simulink model "euler_ZXY_model"  (R2023b)
settings: Solver=FixedStepAuto  StartTime=0.0  StopTime=fs  FixedStep=ts  MaxStep=1e-4  RelTol=1e-3
undefined symbols (not defined in the file): alpha, alpha_1, alpha_2, alpha_d, e1, e2, e3, eta_0, eta_dot_0, f_max, g, gamma, gamma_d, gamma_e, gamma_u, gamma_x, gamma_x1, gamma_x2, J, k_3, k_beta, k_d_gamma, K_p, k_p_gamma, k_R, m, p_0, p_d_0, p_dot_0, p_dot_zmax, r, ts, y_c, z_c, z_dot_max, z_max
libraries: eeGeneralControl x8, slctrl_constraint x6, simulink x2, rbm3d x1, simulink_extras x1
(part 1 of 2)
settings Model: Creator=mori_keigo  LastModifiedBy=mori_keigo

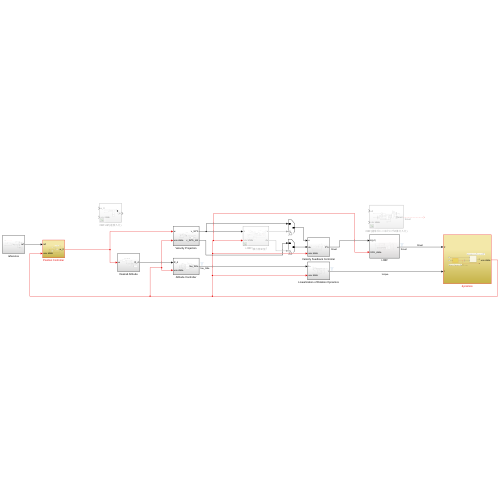
[thumbnail: Simulink's stored preview of the top-level diagram]
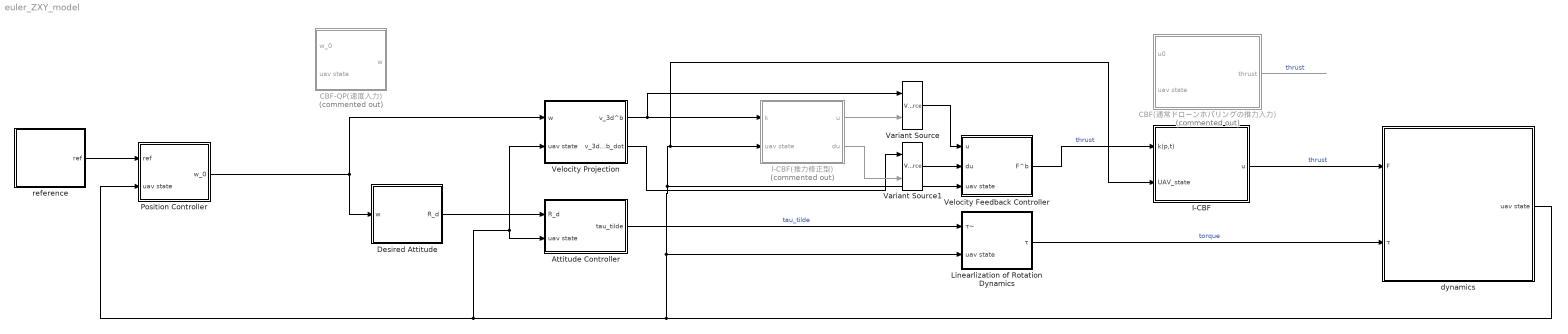
== system euler_ZXY_model ==
  Attitude Controller : Subsystem
  CBF(通常ドローンホバリングの推力入力) : Subsystem  Commented=on
  CBF-QP(速度入力) : Subsystem  Commented=on
  Desired Attitude : Subsystem
  I-CBF : Subsystem
  I-CBF(推力修正型) : Subsystem  Commented=on
  Linearlization of Rotation Dynamics : Subsystem
  Position Controller : Subsystem
  Variant Source : VariantSource
  Variant Source1 : VariantSource
  Velocity Feedback Controller : Subsystem
  Velocity Projection : Subsystem
  dynamics : Subsystem
  reference : Subsystem
  wires:
  Attitude Controller/1(tau_tilde) -> Linearlization of Rotation Dynamics/1(τ~)  "tau_tilde"
  Linearlization of Rotation Dynamics/1(τ) -> dynamics/2(τ)  "torque"
  Desired Attitude/1(R_d) -> Attitude Controller/1(R_d)
  reference/1(ref) -> Position Controller/1(ref)
  Velocity Feedback Controller/1(F^b) -> I-CBF/1(k(p,t))  "thrust"
  Position Controller/1(w_0) -> Desired Attitude/1(w), Velocity Projection/1(w)
  Velocity Projection/1(v_3d^b) -> Variant Source/1, I-CBF(推力修正型)/1(k)
  dynamics/1(uav state) -> I-CBF/2(UAV_state), I-CBF(推力修正型)/2(uav state), Velocity Feedback Controller/3(uav state), Linearlization of Rotation Dynamics/2(uav state), Velocity Projection/2(uav state), Attitude Controller/2(uav state), Position Controller/2(uav state)
  I-CBF(推力修正型)/1(u) -> Variant Source/2
  Velocity Projection/2(v_3d^b_dot) -> Variant Source1/1
  I-CBF(推力修正型)/2(du) -> Variant Source1/2
  Variant Source1/1 -> Velocity Feedback Controller/2(du)
  Variant Source/1 -> Velocity Feedback Controller/1(u)
  I-CBF/1(u) -> dynamics/1(F)  "thrust"
  CBF(通常ドローンホバリングの推力入力)/1(thrust) -> ?  "thrust"

== system euler_ZXY_model/Attitude Controller ==
  R_d : Inport
  Bus Element In1 : Inport  Port=2  PortName=uav state  Element=rotation.R_SO(2)
  Bus Element In2 : Inport  Port=2  PortName=uav state  Element=rotation.angle
  Bus Element In3 : Inport  Port=2  PortName=uav state  Element=rotation.velocity
  Constant : Constant  Value=0
  Selector : Selector  InputPortWidth=3  IndexOptions=Index vector (dialog)  Indices=[3]  OutputSizes=1
  Selector1 : Selector  InputPortWidth=3  IndexOptions=Index vector (dialog)  Indices=[3]  OutputSizes=1
  Selector2 : Selector  InputPortWidth=3  IndexOptions=Index vector (dialog)  Indices=[2]  OutputSizes=1
  Vector Concatenate : Concatenate  NumInputs=3
  beta_controller : Subsystem
  gamma_controller : Subsystem
  tau_tilde : Outport
  wires:
  beta_controller/1(tau_tilde_beta^b) -> Vector Concatenate/2
  gamma_controller/1(tau_tilde_gamma^b) -> Vector Concatenate/3
  Constant/1 -> Vector Concatenate/1
  Vector Concatenate/1 -> tau_tilde/1
  Bus Element In1/1 -> beta_controller/3(R_SO(2))
  Bus Element In2/1 -> Selector/1, Selector2/1
  Bus Element In3/1 -> Selector1/1
  Selector/1 -> gamma_controller/1(gamma)
  Selector1/1 -> gamma_controller/2(gamma_dot)
  Selector2/1 -> beta_controller/1(beta_dot)
  R_d/1 -> beta_controller/2(R_d)

== system euler_ZXY_model/CBF(通常ドローンホバリングの推力入力) ==
  u0 : Inport
  uav state : Inport  Port=2
  Bus Selector : BusSelector  OutputSignals=translation.position,translation.velocity,rotation.R,translation.lambda_1
  Constant : Constant  Value=0
  Constant1 : Constant  Value=0
  Constant2 : Constant  Value=0
  Constraint Enforcement : slctrl_constraint/Constraint Enforcement  nc=1  nu=1  c=0  external_c=on  external_umax=off  external_umin=on  Ts=0.1  maxiter=200  tol=1e-6  output_exitflag=on  relax_c=off  relax_u=off
      settings: LibrarySourceBlock=slctrlblks/Constraint Control/Constraint Enforcement
  MATLAB Function : MATLAB Function  TreatAsAtomicUnit=on
  Mux : Mux  Inputs=3
  Scope : Scope
  Scope1 : Scope
  Selector : Selector  InputPortWidth=3  IndexOptions=Index vector (dialog)  Indices=3  OutputSizes=1
  Selector1 : Selector  InputPortWidth=3  IndexOptions=Index vector (dialog)  Indices=3  OutputSizes=1
  Selector2 : Selector  InputPortWidth=3  IndexOptions=Index vector (dialog)  Indices=3  OutputSizes=1
  thrust : Outport
  wires:
  MATLAB Function/3(c) -> Constraint Enforcement/4
  MATLAB Function/2(gx) -> Constraint Enforcement/3
  MATLAB Function/1(fx) -> Constraint Enforcement/2
  uav state/1 -> Bus Selector/1
  Constant/1 -> Constraint Enforcement/5
  Bus Selector/3 -> MATLAB Function/3(rot)  "<R>"
  Bus Selector/4 -> MATLAB Function/4(lambda1)  "<lambda_1>"
  Constant2/1 -> Mux/2
  Constant1/1 -> Mux/1
  Constraint Enforcement/1 -> Scope1/1, Mux/3
  Mux/1 -> thrust/1
  Bus Selector/1 -> Selector/1  "<position>"
  Selector/1 -> MATLAB Function/1(z)
  Bus Selector/2 -> Selector1/1  "<velocity>"
  Selector1/1 -> MATLAB Function/2(z_dot)
  u0/1 -> Selector2/1
  Selector2/1 -> Constraint Enforcement/1
  Constraint Enforcement/2 -> Scope/1

== system euler_ZXY_model/CBF-QP(速度入力) ==
  w_0 : Inport
  In Bus Element : Inport  Port=2  PortName=uav state  Element=translation.position
  In Bus Element1 : Inport  Port=2  PortName=uav state  Element=rotation.angle
  Demux : Demux  Outputs=2
  ECBF-QP : Subsystem  Commented=on
  ECBF-QP_rengo_ver. : Subsystem
  ECBF-QP_z_only : Subsystem  Commented=on
  Scope : Scope
  Scope1 : Scope
  Scope2 : Scope
  Variant Source : VariantSource
  w : Outport
  wires:
  In Bus Element1/1 -> ECBF-QP_rengo_ver./3(eta)
  In Bus Element/1 -> ECBF-QP_rengo_ver./2(p)
  ECBF-QP_rengo_ver./1(Out1) -> Variant Source/2
  w_0/1 -> ECBF-QP_rengo_ver./1(w0), Variant Source/1
  Variant Source/1 -> Demux/1, Scope/1, w/1
  Demux/1 -> Scope2/1
  Demux/2 -> Scope1/1

== system euler_ZXY_model/Desired Attitude ==
  note: $R_d = \left [ (-1)^{\^} \frac{u}{||u||} \quad \frac{u}{||u||} \right ]$
  w : Inport
  Acos : Trigonometry  Operator=asin
  Display : Display
  Mux : Mux  Inputs=3
  Selector1 : Selector  NumberOfDimensions=2  InputPortWidth=3  IndexOptions=Index vector (dialog),Index vector (dialog)  Indices=[2],[1]  OutputSizes=1,1
  Terminator : Terminator
  alpha_d : Constant  Value=alpha_d
  desired attitude : Subsystem
  gamma_d : Constant  Value=gamma_d
  R_d : Outport
  wires:
  w/1 -> desired attitude/1(w)
  alpha_d/1 -> Mux/1
  Acos/1 -> Mux/2
  Selector1/1 -> Acos/1
  gamma_d/1 -> Mux/3
  Mux/1 -> Terminator/1, Display/1  "desired_attitude"
  desired attitude/1(R_d) -> Selector1/1, R_d/1

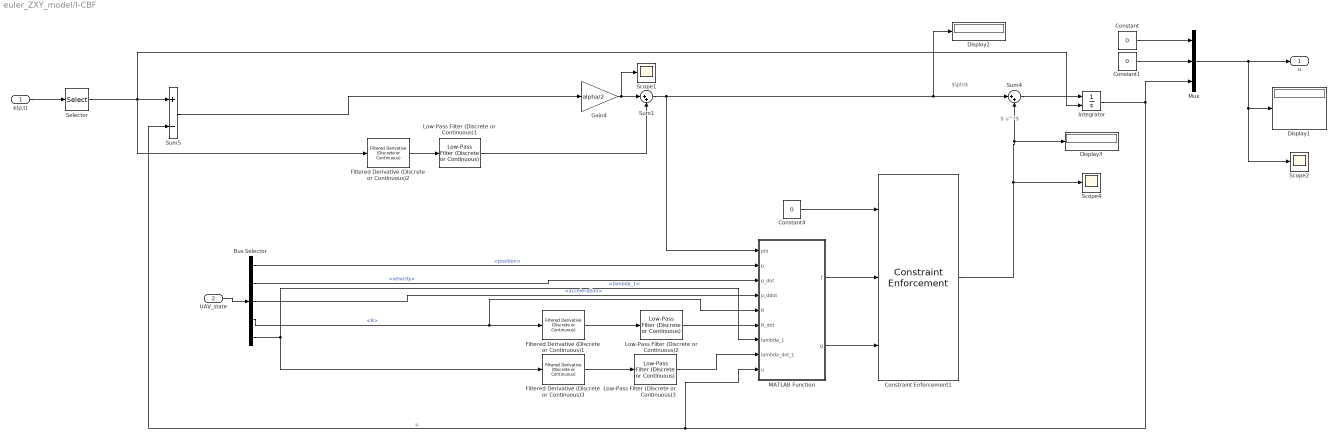
== system euler_ZXY_model/I-CBF ==
  note: $\nu^*$
  note: $\phi$
  k(p,t) : Inport
  UAV_state : Inport  Port=2
  Bus Selector : BusSelector  OutputSignals=translation.position,translation.velocity,translation.acceleration,rotation.R,translation.lambda_1
  Constant : Constant  Value=0
  Constant1 : Constant  Value=0
  Constant4 : Constant  Value=0
  Constraint Enforcement1 : slctrl_constraint/Constraint Enforcement  nc=2  nu=1  c=[0;0]  external_c=off  external_umax=off  external_umin=off  Ts=ts  maxiter=200  tol=1e-6  output_exitflag=on  relax_c=off  relax_u=off
      settings: LibrarySourceBlock=slctrlblks/Constraint Control/Constraint Enforcement
  Display1 : Display
  Display2 : Display
  Display3 : Display
  Filtered Derivative (Discrete or Continuous)1 : eeGeneralControl/Filtered Derivative (Discrete or Continuous)  K=1  T=0.1  B=inf  A=-inf  minRatio=10  init_option=Inherited from block input  x0=0  Ts=-1
      settings: LibrarySourceBlock=|
      | ee_sl_lib/General Control/Filtered Derivative
      | (Discrete or Continuous)
  Filtered Derivative (Discrete or Continuous)2 : eeGeneralControl/Filtered Derivative (Discrete or Continuous)  K=1  T=0.1  B=inf  A=-inf  minRatio=10  init_option=Inherited from block input  x0=0  Ts=-1
      settings: LibrarySourceBlock=|
      | ee_sl_lib/General Control/Filtered Derivative
      | (Discrete or Continuous)
  Filtered Derivative (Discrete or Continuous)3 : eeGeneralControl/Filtered Derivative (Discrete or Continuous)  K=1  T=0.1  B=inf  A=-inf  minRatio=10  init_option=Inherited from block input  x0=0  Ts=-1
      settings: LibrarySourceBlock=|
      | ee_sl_lib/General Control/Filtered Derivative
      | (Discrete or Continuous)
  Gain4 : Gain  Gain=alpha/2
  Integrator : Integrator  InitialConditionSource=external  InitialCondition=5
  Low-Pass Filter (Discrete or Continuous)1 : eeGeneralControl/Low-Pass Filter (Discrete or Continuous)  K=1  T=0.5  B=inf  A=-inf  init_option=Inherited from block input  x0=0  Ts=-1
  Low-Pass Filter (Discrete or Continuous)2 : eeGeneralControl/Low-Pass Filter (Discrete or Continuous)  K=1  T=0.5  B=inf  A=-inf  init_option=Inherited from block input  x0=0  Ts=-1
  Low-Pass Filter (Discrete or Continuous)3 : eeGeneralControl/Low-Pass Filter (Discrete or Continuous)  K=1  T=0.5  B=inf  A=-inf  init_option=Inherited from block input  x0=0  Ts=-1
  MATLAB Function : MATLAB Function  TreatAsAtomicUnit=on
  Mux : Mux  Inputs=3
  Scope1 : Scope
  Scope2 : Scope
  Scope4 : Scope
  Selector : Selector  InputPortWidth=3  IndexOptions=Index vector (dialog)  Indices=3  OutputSizes=1
  Sum1 : Sum  Inputs=|++
  Sum4 : Sum  Inputs=|++
  Sum5 : Sum  Inputs=+-
  u : Outport
  wires:
  UAV_state/1 -> Bus Selector/1
  Sum4/1 -> Integrator/1
  Constraint Enforcement1/1 -> Sum4/2, Display3/1, Scope4/1
  Sum1/1 -> MATLAB Function/1(phi), Display2/1, Sum4/1
  Gain4/1 -> Scope1/1, Sum1/1
  Sum5/1 -> Gain4/1
  Bus Selector/2 -> MATLAB Function/3(p_dot)  "<velocity>"
  Bus Selector/3 -> MATLAB Function/4(p_ddot)  "<acceleration>"
  Constant4/1 -> Constraint Enforcement1/1
  MATLAB Function/1(f) -> Constraint Enforcement1/2
  MATLAB Function/2(g) -> Constraint Enforcement1/3
  Bus Selector/4 -> Filtered Derivative (Discrete or Continuous)1/1, MATLAB Function/5(R)  "<R>"
  Bus Selector/1 -> MATLAB Function/2(p)  "<position>"
  Integrator/1 -> MATLAB Function/9(u), Sum5/2, Mux/3  "u"
  Bus Selector/5 -> MATLAB Function/7(lambda_1), Filtered Derivative (Discrete or Continuous)3/1  "<lambda_1>"
  k(p,t)/1 -> Selector/1
  Selector/1 -> Integrator/2, Sum5/1, Filtered Derivative (Discrete or Continuous)2/1
  Mux/1 -> Scope2/1, Display1/1, u/1
  Constant1/1 -> Mux/2
  Constant/1 -> Mux/1
  Filtered Derivative (Discrete or Continuous)2/1 -> Low-Pass Filter (Discrete or Continuous)1/1
  Low-Pass Filter (Discrete or Continuous)1/1 -> Sum1/2
  Low-Pass Filter (Discrete or Continuous)2/1 -> MATLAB Function/6(R_dot)
  Filtered Derivative (Discrete or Continuous)1/1 -> Low-Pass Filter (Discrete or Continuous)2/1
  Filtered Derivative (Discrete or Continuous)3/1 -> Low-Pass Filter (Discrete or Continuous)3/1
  Low-Pass Filter (Discrete or Continuous)3/1 -> MATLAB Function/8(lambda_dot_1)

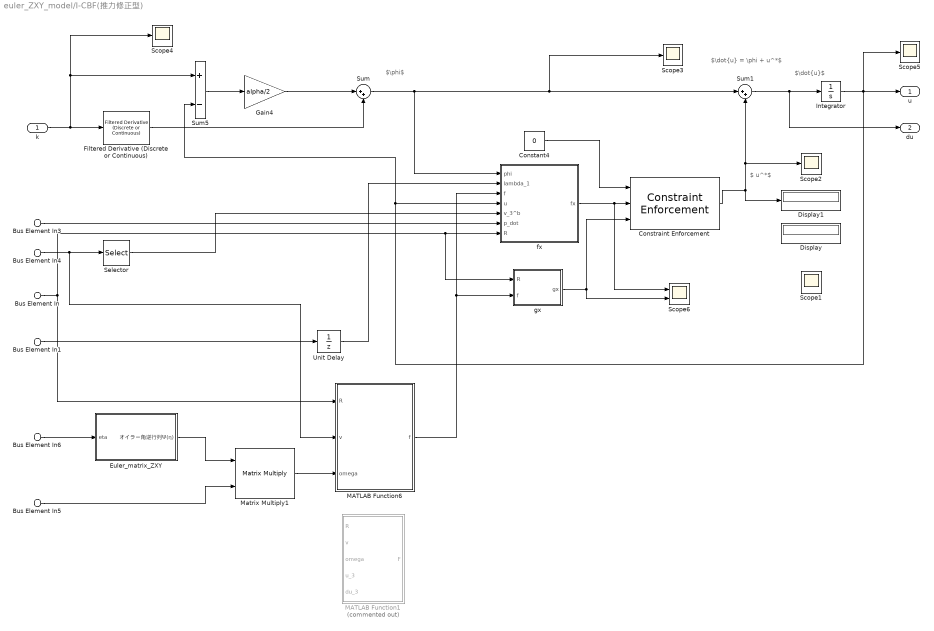
== system euler_ZXY_model/I-CBF(推力修正型) ==
  note: $\dot{u}$
  note: $\dot{u} = \phi + \nu^*$
  note: $\phi$
  note: $\nu^*$
  k : Inport
  Bus Element In : Inport  Port=2  PortName=uav state  Element=rotation.R
  Bus Element In5 : Inport  Port=2  PortName=uav state  Element=rotation.velocity
  Bus Element In6 : Inport  Port=2  PortName=uav state  Element=rotation.angle
  Bus Element In1 : Inport  Port=2  PortName=uav state  Element=translation.lambda_1
  Bus Element In3 : Inport  Port=2  PortName=uav state  Element=translation.velocity
  Bus Element In4 : Inport  Port=2  PortName=uav state  Element=translation.body_velocity
  Constant4 : Constant  Value=0
  Constraint Enforcement : slctrl_constraint/Constraint Enforcement  nc=1  nu=1  c=0  external_c=off  external_umax=off  external_umin=off  Ts=ts  maxiter=200  tol=1e-6  output_exitflag=on  relax_c=off  relax_u=off
      settings: LibrarySourceBlock=slctrlblks/Constraint Control/Constraint Enforcement
  Display : Display
  Display1 : Display
  Euler_matrix_ZXY : Subsystem
  Filtered Derivative (Discrete or Continuous) : eeGeneralControl/Filtered Derivative (Discrete or Continuous)  K=1  T=0.1  B=inf  A=-inf  minRatio=10  init_option=Inherited from block input  x0=0  Ts=-1
      settings: LibrarySourceBlock=|
      | ee_sl_lib/General Control/Filtered Derivative
      | (Discrete or Continuous)
  Gain4 : Gain  Gain=alpha/2
  Integrator : Integrator
  MATLAB Function1 : MATLAB Function  Commented=on  TreatAsAtomicUnit=on
  MATLAB Function6 : MATLAB Function  TreatAsAtomicUnit=on
  Matrix Multiply1 : Product  Multiplication=Matrix(*)
  Scope{1..5} (5 alike) : Scope
  Scope6 : Scope  NumInputPorts=2
  Selector : Selector  InputPortWidth=3  IndexOptions=Index vector (dialog)  Indices=3  OutputSizes=1
  Sum : Sum  Inputs=|++
  Sum1 : Sum  Inputs=|++
  Sum5 : Sum  Inputs=+-
  Unit Delay : UnitDelay  SampleTime=-1  HasFrameUpgradeWarning=on
  fx : Subsystem
  gx : Subsystem
  u : Outport
  du : Outport  Port=2
  wires:
  Integrator/1 -> Scope5/1, u/1, Sum5/2, fx/4(u)
  Constraint Enforcement/1 -> Sum1/2, Scope2/1, Display1/1
  Sum/1 -> fx/1(phi), Scope3/1, Sum1/1
  Gain4/1 -> Sum/1
  Sum5/1 -> Gain4/1
  Constant4/1 -> Constraint Enforcement/1
  ? -> Scope1/1, Display/1
  Sum1/1 -> du/1, Integrator/1
  fx/1(fx) -> Scope6/1, Constraint Enforcement/2
  gx/1(gx) -> Constraint Enforcement/3, Scope6/2
  k/1 -> Filtered Derivative (Discrete or Continuous)/1, Scope4/1, Sum5/1
  Filtered Derivative (Discrete or Continuous)/1 -> Sum/2
  Bus Element In/1 -> gx/1(R), fx/7(R), MATLAB Function6/1(R)
  MATLAB Function6/1(f) -> fx/3(f), gx/2(f)
  Bus Element In5/1 -> Matrix Multiply1/2
  Bus Element In6/1 -> Euler_matrix_ZXY/1(eta)
  Euler_matrix_ZXY/1(オイラー角逆行列Ψ(η)) -> Matrix Multiply1/1
  Matrix Multiply1/1 -> MATLAB Function6/3(omega)
  Bus Element In4/1 -> MATLAB Function6/2(v), Selector/1
  Selector/1 -> fx/5(v_3^b)
  Bus Element In3/1 -> fx/6(p_dot)
  Bus Element In1/1 -> Unit Delay/1
  Unit Delay/1 -> fx/2(lambda_1)

== system euler_ZXY_model/Linearlization of Rotation Dynamics ==
  τ~ : Inport
  Bus Element In1 : Inport  Port=2  PortName=uav state  Element=rotation.Psi
  Bus Element In2 : Inport  Port=2  PortName=uav state  Element=rotation.lambda_3
  Bus Element In3 : Inport  Port=2  PortName=uav state  Element=rotation.velocity
  Constant : Constant  Value=J  VectorParams1D=off
  Constant1 : Constant  Value=e1
  Product : Product  Inputs=3  Multiplication=Matrix(*)
  Product1 : Product  Inputs=/  Multiplication=Matrix(*)
  Product2 : Product  Inputs=3  Multiplication=Matrix(*)
  Product3 : Product  Multiplication=Matrix(*)
  Scope : Scope
  Sum : Sum  Inputs=|+++
  Transpose1 : Math  Operator=transpose
  Unit Delay : UnitDelay  SampleTime=-1  HasFrameUpgradeWarning=on
  τ : Outport
  wires:
  τ~/1 -> Scope/1, Product/3
  Constant/1 -> Product/1
  Product/1 -> Sum/1
  Product2/1 -> Sum/2
  Sum/1 -> τ/1
  Bus Element In1/1 -> Transpose1/1, Product/2
  Transpose1/1 -> Product1/1
  Constant1/1 -> Product3/1
  Product3/1 -> Sum/3
  Bus Element In2/1 -> Unit Delay/1
  Unit Delay/1 -> Product3/2
  Product1/1 -> Product2/1
  [C] -> Product2/2
  Bus Element In3/1 -> Product2/3

== system euler_ZXY_model/Position Controller ==
  note: $w_0 = - K_p ~ p_e + \dot{p}_d$
  Bus Element In : Inport  PortName=ref  Element=position
  Bus Element In1 : Inport  PortName=ref  Element=velocity
  In Bus Element : Inport  Port=2  PortName=uav state  Element=translation.position
  Constant : Constant  Value=K_p
  Matrix Multiply : Product  Multiplication=Matrix(*)
  Selector : Selector  InputPortWidth=3  IndexOptions=Index vector (dialog)  Indices=[2 3]  OutputSizes=1
  Sum : Sum  Inputs=|+-
  Sum1 : Sum  Inputs=|++
  w_0 : Outport
  wires:
  Bus Element In/1 -> Sum/1
  Matrix Multiply/1 -> Sum1/1
  Constant/1 -> Matrix Multiply/1
  Sum/1 -> Matrix Multiply/2
  Sum1/1 -> w_0/1
  Bus Element In1/1 -> Sum1/2
  In Bus Element/1 -> Selector/1
  Selector/1 -> Sum/2

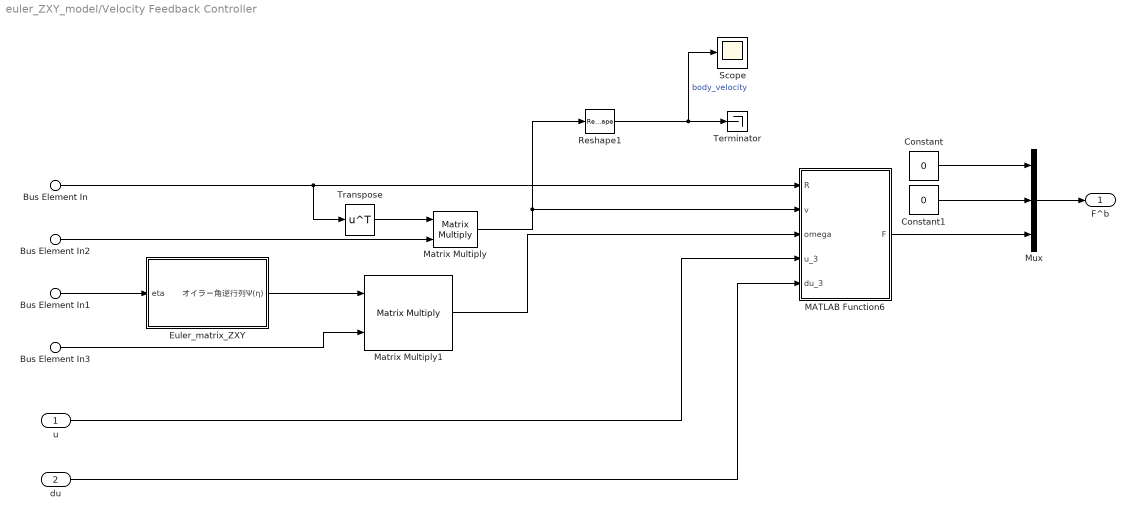
== system euler_ZXY_model/Velocity Feedback Controller ==
  u : Inport
  du : Inport  Port=2
  Bus Element In3 : Inport  Port=3  PortName=uav state  Element=rotation.velocity
  Bus Element In1 : Inport  Port=3  PortName=uav state  Element=rotation.angle
  Bus Element In : Inport  Port=3  PortName=uav state  Element=rotation.R
  Bus Element In2 : Inport  Port=3  PortName=uav state  Element=translation.velocity
  Constant : Constant  Value=0
  Constant1 : Constant  Value=0
  Euler_matrix_ZXY : Subsystem
  MATLAB Function6 : MATLAB Function  TreatAsAtomicUnit=on
  Matrix Multiply : Product  Multiplication=Matrix(*)
  Matrix Multiply1 : Product  Multiplication=Matrix(*)
  Mux : Mux  Inputs=3
  Reshape1 : Reshape
  Scope : Scope
  Terminator : Terminator
  Transpose : Math  Operator=transpose
  F^b : Outport
  wires:
  u/1 -> MATLAB Function6/4(u_3)
  Transpose/1 -> Matrix Multiply/1
  Bus Element In2/1 -> Matrix Multiply/2
  Bus Element In/1 -> MATLAB Function6/1(R), Transpose/1
  Matrix Multiply1/1 -> MATLAB Function6/3(omega)
  Matrix Multiply/1 -> Reshape1/1, MATLAB Function6/2(v)
  Reshape1/1 -> Scope/1, Terminator/1  "body_velocity"
  Bus Element In3/1 -> Matrix Multiply1/2
  Euler_matrix_ZXY/1(オイラー角逆行列Ψ(η)) -> Matrix Multiply1/1
  Bus Element In1/1 -> Euler_matrix_ZXY/1(eta)
  MATLAB Function6/1(F) -> Mux/3
  Mux/1 -> F^b/1
  Constant1/1 -> Mux/2
  Constant/1 -> Mux/1
  du/1 -> MATLAB Function6/5(du_3)

== system euler_ZXY_model/Velocity Projection ==
  note: $v_z = u^T Re_2$
  w : Inport
  In Bus Element : Inport  Port=2  PortName=uav state  Element=rotation.R_SO(2)
  Constant : Constant  Value=[0;1]  VectorParams1D=off
  Filtered Derivative (Discrete or Continuous)2 : eeGeneralControl/Filtered Derivative (Discrete or Continuous)  K=1  T=0.1  B=inf  A=-inf  minRatio=10  init_option=Inherited from block input  x0=0  Ts=-1
      settings: LibrarySourceBlock=|
      | ee_sl_lib/General Control/Filtered Derivative
      | (Discrete or Continuous)
  Matrix Multiply : Product  Inputs=3  Multiplication=Matrix(*)
  Transpose : Math  Operator=transpose
  v_3d^b : Outport
  v_3d^b_dot : Outport  Port=2
  wires:
  In Bus Element/1 -> Matrix Multiply/2
  Transpose/1 -> Matrix Multiply/1
  Matrix Multiply/1 -> Filtered Derivative (Discrete or Continuous)2/1, v_3d^b/1
  w/1 -> Transpose/1
  Constant/1 -> Matrix Multiply/3
  Filtered Derivative (Discrete or Continuous)2/1 -> v_3d^b_dot/1

== system euler_ZXY_model/dynamics ==
  note: $m \ddot{p} + mg e_3 + \lambda_1 A^T + \lambda_2 e_1 = RF^b$
  note: $M(\eta) \ddot{\eta} + C(\eta,\dot{\eta}) \dot{\eta} = \Psi(\eta)^T \tau^b - \lambda_3 e_1$
  F : Inport
  τ : Inport  Port=2
  Bus Selector : BusSelector  OutputSignals=angle
  並進方向の運動方程式 : Subsystem
  回転方向の運動方程式 : Subsystem
  Bus Element Out1 : Outport  PortName=uav state  Element=translation
  Bus Element Out : Outport  PortName=uav state  Element=rotation
  wires:
  τ/1 -> 回転方向の運動方程式/1(τ^b)
  F/1 -> 並進方向の運動方程式/1(F_b)
  並進方向の運動方程式/1(translation) -> Bus Element Out1/1
  回転方向の運動方程式/1(attitude_state) -> Bus Selector/1, Bus Element Out/1
  Bus Selector/1 -> 並進方向の運動方程式/2(eta)  "<angle>"

== system euler_ZXY_model/reference ==
  Clock1 : Clock
  Constant : Constant  Value=0.20
  Constant1 : Constant  Value=0
  Constant2 : Constant  Commented=on  Value=0
  Demux : Demux  Outputs=2
  Integrator : Integrator  InitialCondition=p_d_0
  Mux : Mux  Inputs=2
  Mux1 : Mux  Inputs=2
  Terminator : Terminator
  XY Graph : Record  FileSettingsInternal="{\"entries\":[{\"content\":{\"excelSettings\":{\"content\":{},\"type\":\"Streamout.ExcelSettings\"}},\"type\":\"Streamout.FileSettingStorage\",\"uuid\":\"\"}],\"packageUris\":[\"http:\\/\\/schema.mathworks.com\\/mf0\\/streamout_blocks\\/R2020a\"],\"version\":\"1.0\"}"  Layout=[1 1]  SignalsInternal="{\"entries\":[{\"content\":{\"signals\":[{\"content\":{\"blockPath\":[],\"dimensions\":[1],\"domain\":\"\",\"lineColor\":\"#edb120\",\"port\":1,\"signalID\":8,\"signalName\":\"Demux:1\"},\"type\":\"RecordBlkView.Signal\",\"uuid\":\"\"},{\"content\":{\"blockPath\":[],\"dimensions\":[1],\"domain\":\"\",\"lineColor\":\"#7e2f8e\",\"port\":2,\"signalID\":11,\"signalName\":\"Demux:2\"},\"type\":\"RecordBlkView.Signal\",\"uuid\":\"\"}]},\"type\":\"RecordBlkView.InputSignals\",\"uuid\":\"\"}],\"packageUris\":[\"http:\\/\\/schema.mathworks.com\\/mf0\\/streamout_blocks\\/R2020a\"],\"version\":\"1.0\"}"  VisualizationBindings="{\"xyplotplugin\":{\"info\":[{\"series\":[],\"subplotID\":1}]}}"  CompatibilityTag=XY
  y_d_dot : Stateflow chart  TreatAsAtomicUnit=on
  Out Bus Element : Outport  PortName=ref  Element=position
  Out Bus Element1 : Outport  PortName=ref  Element=velocity
  wires:
  Clock1/1 -> y_d_dot/1(t)
  Constant/1 -> Mux/2
  y_d_dot/1(y_d_dot) -> Mux/1
  Mux/1 -> Out Bus Element1/1, Integrator/1
  Demux/1 -> XY Graph/1
  Demux/2 -> XY Graph/2
  Integrator/1 -> Mux1/2, Out Bus Element/1, Demux/1
  Constant1/1 -> Mux1/1
  Mux1/1 -> Terminator/1  "p_d"
  Constant2/1 -> ?

== system euler_ZXY_model/Attitude Controller/beta_controller ==
  beta_dot : Inport
  R_d : Inport  Port=2
  R_SO(2) : Inport  Port=3
  Derivative : Derivative  Commented=on
  Discrete Derivative : simulink/Discrete/Discrete Derivative  gainval=1.0  ICPrevScaledInput=0.0  OutMin=[]  OutMax=[]  OutDataType=fixdt(1, 16)  OutScaling=2^-10  DoSatur=off
  Gain : Gain  Gain=-k_beta
  Scope : Scope
  Scope1 : Scope
  Sum : Sum  Inputs=|+-
  Sum1 : Sum  Inputs=|++
  r_beta : Subsystem
  tau_tilde_beta^b : Outport
  wires:
  beta_dot/1 -> Sum/1
  Gain/1 -> Sum1/1
  Sum1/1 -> Scope1/1, tau_tilde_beta^b/1
  r_beta/1(r_beta) -> Discrete Derivative/1, Sum/2
  Sum/1 -> Scope/1, Gain/1
  Discrete Derivative/1 -> Sum1/2
  R_d/1 -> r_beta/1(R_d)
  R_SO(2)/1 -> r_beta/2(R_SO(2))

== system euler_ZXY_model/Attitude Controller/gamma_controller ==
  gamma : Inport
  gamma_dot : Inport  Port=2
  Constant : Constant  Value=gamma_d
  Derivative : Derivative
  Gain : Gain  Gain=-k_p_gamma
  Gain1 : Gain  Gain=-k_d_gamma
  Sum : Sum  Inputs=|++
  Sum1 : Sum  Inputs=|-+
  Sum2 : Sum  Inputs=|-+
  tau_tilde_gamma^b : Outport
  wires:
  Sum/1 -> tau_tilde_gamma^b/1
  Gain/1 -> Sum/1
  Gain1/1 -> Sum/2
  Constant/1 -> Derivative/1, Sum1/1
  Sum2/1 -> Gain1/1
  Derivative/1 -> Sum2/1
  Sum1/1 -> Gain/1
  gamma/1 -> Sum1/2
  gamma_dot/1 -> Sum2/2

== system euler_ZXY_model/CBF-QP(速度入力)/ECBF-QP ==
  u0 : Inport
  p : Inport  Port=2
  eta : Inport  Port=3
  p_dot : Inport  Port=4
  body_velocity : Inport  Port=5
  eta_dot : Inport  Port=6
  Constraint Enforcement : slctrl_constraint/Constraint Enforcement  nc=1  nu=2  c=0  external_c=on  external_umax=off  external_umin=off  Ts=0.01  maxiter=200  tol=1e-6  output_exitflag=off  relax_c=off  relax_u=off
  Scope : Scope
  Scope1 : Scope
  Subsystem : Subsystem
  c : Subsystem
  gx : Subsystem
  Out1 : Outport
  wires:
  u0/1 -> Constraint Enforcement/1, Scope/1
  p/1 -> Subsystem/1(p), gx/1(p), c/1(p)
  eta/1 -> Subsystem/3(eta), gx/2(eta)
  Subsystem/1(fx) -> Constraint Enforcement/2
  gx/1(gx) -> Constraint Enforcement/3
  c/1(c) -> Constraint Enforcement/4
  Constraint Enforcement/1 -> Scope1/1, Out1/1
  p_dot/1 -> Subsystem/2(p_dot), c/2(p_dot)
  body_velocity/1 -> Subsystem/4(body_velocity)
  eta_dot/1 -> Subsystem/5(eta_dot)

== system euler_ZXY_model/CBF-QP(速度入力)/ECBF-QP_rengo_ver. ==
  w0 : Inport
  p : Inport  Port=2
  eta : Inport  Port=3
  Constraint Enforcement : slctrl_constraint/Constraint Enforcement  nc=1  nu=2  c=0  external_c=on  external_umax=off  external_umin=off  Ts=0.01  maxiter=200  tol=1e-6  output_exitflag=off  relax_c=off  relax_u=off
  Scope : Scope
  Scope1 : Scope
  c : Subsystem
  fx : Constant  Value=0  VectorParams1D=off
  gx : Subsystem
  Out1 : Outport
  wires:
  w0/1 -> Scope/1, Constraint Enforcement/1
  p/1 -> c/1(p), gx/1(p)
  eta/1 -> gx/2(eta), c/2(eta)
  fx/1 -> Constraint Enforcement/2
  gx/1(gx) -> Constraint Enforcement/3
  c/1(c) -> Constraint Enforcement/4
  Constraint Enforcement/1 -> Scope1/1, Out1/1

== system euler_ZXY_model/CBF-QP(速度入力)/ECBF-QP_z_only ==
  u0 : Inport
  p : Inport  Port=2
  eta : Inport  Port=3
  p_dot : Inport  Port=4
  body_velocity : Inport  Port=5
  eta_dot : Inport  Port=6
  Constraint Enforcement : slctrl_constraint/Constraint Enforcement  nc=1  nu=2  c=0  external_c=on  external_umax=off  external_umin=off  Ts=0.01  maxiter=200  tol=1e-6  output_exitflag=off  relax_c=off  relax_u=off
  Scope : Scope
  Scope1 : Scope
  Subsystem : Subsystem
  c : Subsystem
  gx : Subsystem
  Out1 : Outport
  wires:
  u0/1 -> Constraint Enforcement/1, Scope/1
  p/1 -> c/1(p)
  eta/1 -> Subsystem/1(eta), gx/1(eta)
  Subsystem/1(fx) -> Constraint Enforcement/2
  gx/1(gx) -> Constraint Enforcement/3
  c/1(c) -> Constraint Enforcement/4
  Constraint Enforcement/1 -> Scope1/1, Out1/1
  p_dot/1 -> c/2(p_dot)
  body_velocity/1 -> Subsystem/2(body_velocity)
  eta_dot/1 -> Subsystem/3(eta_dot)

== system euler_ZXY_model/Desired Attitude/desired attitude ==
  w : Inport
  (-1)^ : Constant  Value=[0 1; -1 0]  VectorParams1D=off
  Divide : Product  Inputs=*/
  Dot Product : DotProduct  OutDataTypeStr=Inherit: Inherit via internal rule
  Matrix Concatenate : Concatenate  Mode=Multidimensional array  ConcatenateDimension=2
  Matrix Multiply : Product  Multiplication=Matrix(*)
  Square Root : Sqrt
  R_d : Outport
  wires:
  Dot Product/1 -> Square Root/1
  w/1 -> Divide/1, Dot Product/2, Dot Product/1
  Square Root/1 -> Divide/2
  Matrix Concatenate/1 -> R_d/1
  Divide/1 -> Matrix Concatenate/2, Matrix Multiply/2
  (-1)^/1 -> Matrix Multiply/1
  Matrix Multiply/1 -> Matrix Concatenate/1

== system euler_ZXY_model/I-CBF(推力修正型)/Euler_matrix_ZXY ==
  eta : Inport
  Constant : Constant  Value=e2
  Matrix Concatenate4 : Concatenate  NumInputs=3  Mode=Multidimensional array  ConcatenateDimension=2
  Psi_*1 : Subsystem
  Psi_*2 : Subsystem
  オイラー角逆行列Ψ(η) : Outport  VectorParamsAs1DForOutWhenUnconnected=off
  wires:
  eta/1 -> Psi_*1/1(eta), Psi_*2/1(eta)
  Matrix Concatenate4/1 -> オイラー角逆行列Ψ(η)/1
  Psi_*2/1(Out1) -> Matrix Concatenate4/2
  Psi_*1/1(Out1) -> Matrix Concatenate4/1
  Constant/1 -> Matrix Concatenate4/3

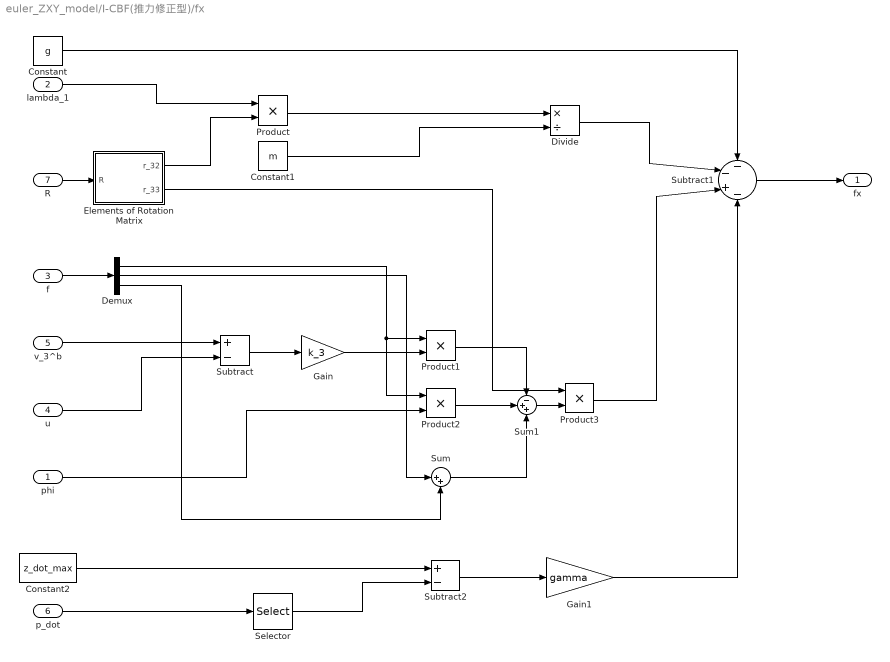
== system euler_ZXY_model/I-CBF(推力修正型)/fx ==
  phi : Inport
  lambda_1 : Inport  Port=2
  f : Inport  Port=3
  u : Inport  Port=4
  v_3^b : Inport  Port=5
  p_dot : Inport  Port=6
  R : Inport  Port=7
  Constant : Constant  Value=g
  Constant1 : Constant  Value=m
  Constant2 : Constant  Value=z_dot_max
  Demux : Demux  Outputs=3
  Divide : Product  Inputs=*/
  Elements of Rotation Matrix : Subsystem
  Gain : Gain  Gain=k_3
  Gain1 : Gain  Gain=gamma
  Product{,1..3} (4 alike) : Product
  Selector : Selector  InputPortWidth=3  IndexOptions=Index vector (dialog)  Indices=3  OutputSizes=1
  Subtract : Sum  Inputs=+-
  Subtract1 : Sum  Inputs=--+-
  Subtract2 : Sum  Inputs=+-
  Sum : Sum  Inputs=|++
  Sum1 : Sum  Inputs=-++
  fx : Outport
  wires:
  Constant/1 -> Subtract1/1
  lambda_1/1 -> Product/1
  Product/1 -> Divide/1
  Constant1/1 -> Divide/2
  Divide/1 -> Subtract1/2
  Subtract1/1 -> fx/1
  v_3^b/1 -> Subtract/1
  u/1 -> Subtract/2
  Subtract/1 -> Gain/1
  Gain/1 -> Product1/2
  phi/1 -> Product2/2
  f/1 -> Demux/1
  Demux/1 -> Product2/1, Product1/1
  Demux/2 -> Sum/1
  Demux/3 -> Sum/2
  Product1/1 -> Sum1/1
  Product2/1 -> Sum1/2
  Sum/1 -> Sum1/3
  Sum1/1 -> Product3/2
  Constant2/1 -> Subtract2/1
  Subtract2/1 -> Gain1/1
  Product3/1 -> Subtract1/3
  Gain1/1 -> Subtract1/4
  p_dot/1 -> Selector/1
  Selector/1 -> Subtract2/2
  R/1 -> Elements of Rotation Matrix/1(R)
  Elements of Rotation Matrix/1(r_32) -> Product/2
  Elements of Rotation Matrix/2(r_33) -> Product3/1

== system euler_ZXY_model/I-CBF(推力修正型)/gx ==
  R : Inport
  f : Inport  Port=2
  Elements of Rotation Matrix : Subsystem
  Product : Product
  Selector : Selector  InputPortWidth=3  IndexOptions=Index vector (dialog)  Indices=1  OutputSizes=1
  gx : Outport
  wires:
  R/1 -> Elements of Rotation Matrix/1(R)
  f/1 -> Selector/1
  Selector/1 -> Product/2
  Product/1 -> gx/1
  Elements of Rotation Matrix/1(r_33) -> Product/1

== system euler_ZXY_model/Velocity Feedback Controller/Euler_matrix_ZXY ==
  eta : Inport
  Constant : Constant  Value=e2
  Matrix Concatenate4 : Concatenate  NumInputs=3  Mode=Multidimensional array  ConcatenateDimension=2
  Psi_*1 : Subsystem
  Psi_*2 : Subsystem
  オイラー角逆行列Ψ(η) : Outport  VectorParamsAs1DForOutWhenUnconnected=off
  tag scope: euler_matrix_inv=global
  wires:
  eta/1 -> Psi_*1/1(eta), Psi_*2/1(eta)
  Matrix Concatenate4/1 -> [euler_matrix_inv], オイラー角逆行列Ψ(η)/1
  Psi_*2/1(Out1) -> Matrix Concatenate4/2
  Psi_*1/1(Out1) -> Matrix Concatenate4/1
  Constant/1 -> Matrix Concatenate4/3

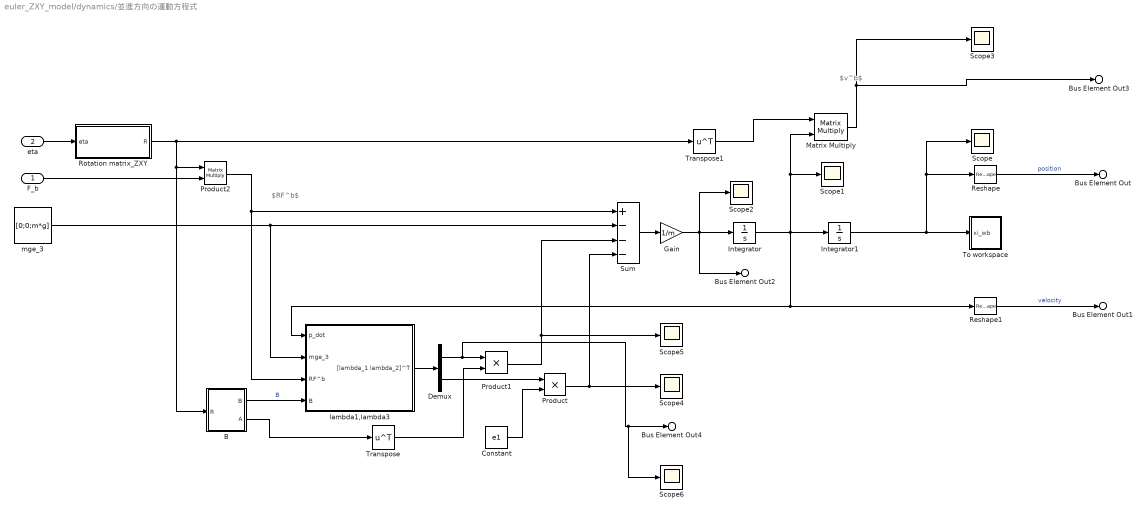
== system euler_ZXY_model/dynamics/並進方向の運動方程式 ==
  note: $v^b$
  note: $RF^b$
  F_b : Inport
  eta : Inport  Port=2
  B : Subsystem
  Constant : Constant  Value=e1
  Demux : Demux  Outputs=2
  Gain : Gain  Gain=1/m
  Integrator : Integrator  InitialCondition=p_dot_0
  Integrator1 : Integrator  InitialCondition=p_0
  Matrix Multiply : Product  Multiplication=Matrix(*)
  Product : Product
  Product1 : Product
  Product2 : Product  Multiplication=Matrix(*)
  Reshape : Reshape
  Reshape1 : Reshape
  Rotation matrix_ZXY : Subsystem
  Scope{,1..6} (7 alike) : Scope
  Sum : Sum  Inputs=+---
  To workspace : Subsystem
  Transpose : Math  Operator=transpose
  Transpose1 : Math  Operator=transpose
  lambda1,lambda3 : Subsystem
  mge_3 : Constant  Value=[0;0;m*g]  VectorParams1D=off
  Bus Element Out : Outport  PortName=translation  Element=position
  Bus Element Out1 : Outport  PortName=translation  Element=velocity
  Bus Element Out2 : Outport  PortName=translation  Element=acceleration
  Bus Element Out3 : Outport  PortName=translation  Element=body_velocity
  Bus Element Out4 : Outport  PortName=translation  Element=lambda_1
  wires:
  Integrator1/1 -> Scope/1, Reshape/1, To workspace/1(xi_wb)
  Integrator/1 -> Integrator1/1, Reshape1/1, lambda1,lambda3/1(p_dot), Matrix Multiply/2, Scope1/1
  Product2/1 -> lambda1,lambda3/3(RF^b), Sum/1
  mge_3/1 -> lambda1,lambda3/2(mge_3), Sum/2
  eta/1 -> Rotation matrix_ZXY/1(eta)
  Rotation matrix_ZXY/1(R) -> Transpose1/1, Product2/1, B/1(R)
  F_b/1 -> Product2/2
  Sum/1 -> Gain/1
  Gain/1 -> Scope2/1, Integrator/1, Bus Element Out2/1
  B/1(B) -> lambda1,lambda3/4(B)  "B"
  Product/1 -> Scope4/1, Sum/4
  B/2(A) -> Transpose/1
  Product1/1 -> Sum/3, Scope5/1
  Demux/1 -> Scope6/1, Bus Element Out4/1, Product1/1
  Demux/2 -> Product/1
  lambda1,lambda3/1("[lambda_1 lambda_2]^T") -> Demux/1
  Constant/1 -> Product/2
  Transpose/1 -> Product1/2
  Transpose1/1 -> Matrix Multiply/1
  Matrix Multiply/1 -> Bus Element Out3/1, Scope3/1
  Reshape/1 -> Bus Element Out/1  "position"
  Reshape1/1 -> Bus Element Out1/1  "velocity"

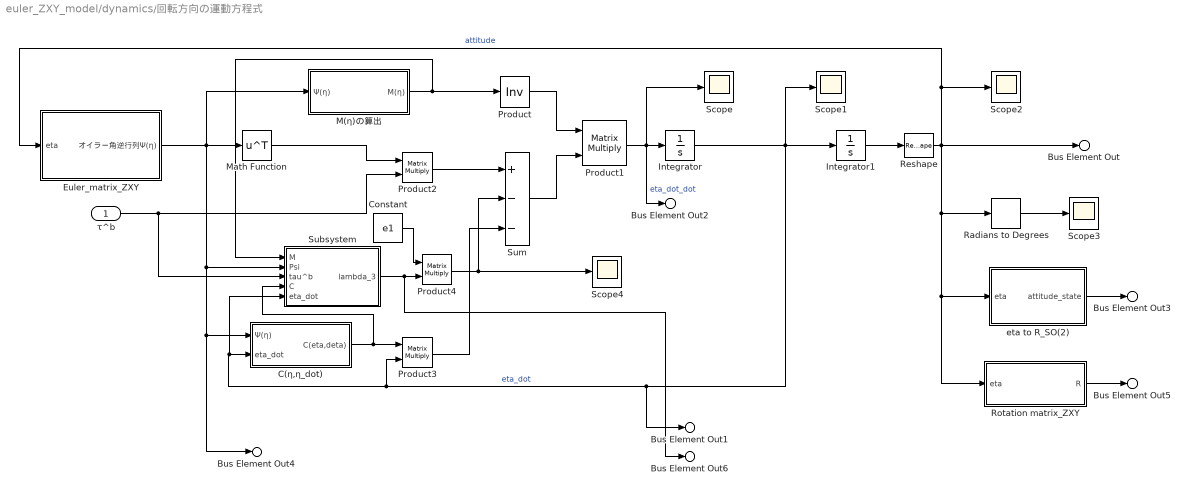
== system euler_ZXY_model/dynamics/回転方向の運動方程式 ==
  τ^b : Inport
  C(η,η_dot) : Subsystem
  Constant : Constant  Value=e1
  Euler_matrix_ZXY : Subsystem
  Integrator : Integrator  InitialCondition=eta_dot_0
  Integrator1 : Integrator  InitialCondition=eta_0
  M(η)の算出 : Subsystem
  Math Function : Math  Operator=transpose  SignedPower=on
  Product : Product  Inputs=/  Multiplication=Matrix(*)
  Product{1..4} (4 alike) : Product  Multiplication=Matrix(*)
  Radians to Degrees : simulink_extras/Transformations/Radians to Degrees
  Reshape : Reshape
  Rotation matrix_ZXY : Subsystem
  Scope{,1..4} (5 alike) : Scope
  Subsystem : Subsystem
  Sum : Sum  Inputs=+--
  eta to R_SO(2) : Subsystem
  Bus Element Out : Outport  PortName=attitude_state  Element=angle
  Bus Element Out1 : Outport  PortName=attitude_state  Element=velocity
  Bus Element Out2 : Outport  PortName=attitude_state  Element=acceleration
  Bus Element Out3 : Outport  PortName=attitude_state  Element=R_SO(2)
  Bus Element Out4 : Outport  PortName=attitude_state  Element=Psi
  Bus Element Out5 : Outport  PortName=attitude_state  Element=R
  Bus Element Out6 : Outport  PortName=attitude_state  Element=lambda_3
  wires:
  Product/1 -> Product1/1
  M(η)の算出/1(M(η)) -> Subsystem/1(M), Product/1
  τ^b/1 -> Subsystem/3(tau^b), Product2/2
  Product1/1 -> Scope/1, Bus Element Out2/1, Integrator/1  "eta_dot_dot"
  Product2/1 -> Sum/1
  Reshape/1 -> Euler_matrix_ZXY/1(eta), Scope2/1, Bus Element Out/1, Rotation matrix_ZXY/1(eta), eta to R_SO(2)/1(eta), Radians to Degrees/1  "attitude"
  C(η,η_dot)/1(C(eta,deta)) -> Subsystem/4(C), Product3/1
  Sum/1 -> Product1/2
  Integrator/1 -> Scope1/1, Product3/2, Subsystem/5(eta_dot), C(η,η_dot)/2(eta_dot), Bus Element Out1/1, Integrator1/1  "eta_dot"
  Product3/1 -> Sum/3
  Euler_matrix_ZXY/1(オイラー角逆行列Ψ(η)) -> Subsystem/2(Psi), Bus Element Out4/1, C(η,η_dot)/1(Ψ(η)), Math Function/1, M(η)の算出/1(Ψ(η))
  Math Function/1 -> Product2/1
  Radians to Degrees/1 -> Scope3/1
  Product4/1 -> Sum/2, Scope4/1
  eta to R_SO(2)/1(attitude_state) -> Bus Element Out3/1
  Rotation matrix_ZXY/1(R) -> Bus Element Out5/1
  Subsystem/1(lambda_3) -> Bus Element Out6/1, Product4/2
  Constant/1 -> Product4/1
  Integrator1/1 -> Reshape/1

== system euler_ZXY_model/Attitude Controller/beta_controller/r_beta ==
  R_d : Inport
  R_SO(2) : Inport  Port=2
  Discrete Derivative : simulink/Discrete/Discrete Derivative  gainval=1.0  ICPrevScaledInput=0.0  OutMin=[]  OutMax=[]  OutDataType=fixdt(1, 16)  OutScaling=2^-10  DoSatur=off
  Gain : Gain  Gain=k_R
  Gain1 : Gain  Gain=1/2
  R_tilde : Subsystem
  Selector : Selector  NumberOfDimensions=2  InputPortWidth=3  IndexOptions=Index vector (dialog),Index vector (dialog)  Indices=[2],1  OutputSizes=1,1
  Sum : Sum  Inputs=|+-
  Sum1 : Sum  Inputs=|+-
  Transpose : Math  Operator=transpose
  r_beta_d : Subsystem
  r_beta : Outport
  wires:
  r_beta_d/1("r_{beta_d}") -> Sum/1
  Sum/1 -> r_beta/1
  Gain/1 -> Sum/2
  Selector/1 -> Gain/1
  Transpose/1 -> Sum1/2
  R_tilde/1(R_tilde) -> Transpose/1, Sum1/1
  Gain1/1 -> Selector/1
  Sum1/1 -> Gain1/1
  R_d/1 -> R_tilde/1(R_d), Discrete Derivative/1, r_beta_d/1(R_d)
  Discrete Derivative/1 -> r_beta_d/2(R_d_dot)
  R_SO(2)/1 -> R_tilde/2(R)

== system euler_ZXY_model/CBF-QP(速度入力)/ECBF-QP/Subsystem ==
  p : Inport
  p_dot : Inport  Port=2
  eta : Inport  Port=3
  body_velocity : Inport  Port=4
  eta_dot : Inport  Port=5
  Scope : Scope  NumInputPorts=3
  Sum : Sum  Inputs=|+++
  f_x : Subsystem
  f_x1 : Subsystem
  f_x2 : Subsystem
  fx : Outport
  wires:
  p_dot/1 -> f_x1/1(p_dot)
  p/1 -> f_x/1(p), f_x2/1(p)
  eta/1 -> f_x/2(eta), f_x2/2(eta)
  body_velocity/1 -> f_x/3(body_velocity), f_x2/3(body_velocity)
  eta_dot/1 -> f_x2/4(eta_dot), f_x/4(eta_dot)
  f_x2/1(f_x2) -> Scope/2, Sum/2
  f_x1/1(f_x1) -> Scope/1, Sum/1
  f_x/1(f_x3) -> Scope/3, Sum/3
  Sum/1 -> fx/1

== system euler_ZXY_model/CBF-QP(速度入力)/ECBF-QP/c ==
  p : Inport
  p_dot : Inport  Port=2
  Gain : Gain  Gain=alpha_1
  Gain1 : Gain  Gain=alpha_2
  Subsystem : Subsystem
  Sum : Sum  Inputs=|++
  h : Subsystem
  c : Outport
  wires:
  p/1 -> Subsystem/1(p), h/1(p)
  h/1(h) -> Gain/1
  Gain/1 -> Sum/1
  Sum/1 -> c/1
  Subsystem/1(h_dot) -> Gain1/1
  Gain1/1 -> Sum/2
  p_dot/1 -> Subsystem/2(p_dot)

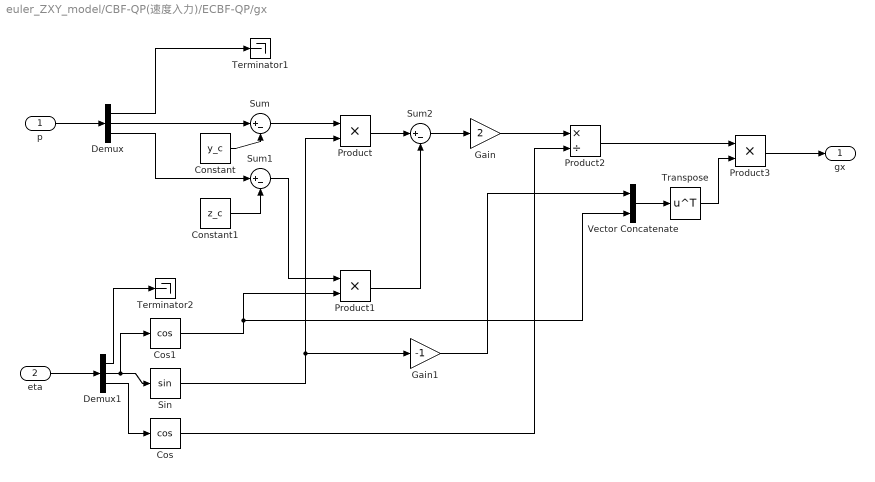
== system euler_ZXY_model/CBF-QP(速度入力)/ECBF-QP/gx ==
  p : Inport
  eta : Inport  Port=2
  Constant : Constant  Value=y_c
  Constant1 : Constant  Value=z_c
  Cos : Trigonometry  Operator=cos
  Cos1 : Trigonometry  Operator=cos
  Demux : Demux  Outputs=3
  Demux1 : Demux  Outputs=3
  Gain : Gain  Gain=2
  Gain1 : Gain  Gain=-1
  Product : Product
  Product1 : Product
  Product2 : Product  Inputs=*/
  Product3 : Product
  Sin : Trigonometry
  Sum : Sum  Inputs=|+-
  Sum1 : Sum  Inputs=|+-
  Sum2 : Sum  Inputs=|+-
  Terminator1 : Terminator
  Terminator2 : Terminator
  Transpose : Math  Operator=transpose
  Vector Concatenate : Concatenate
  gx : Outport
  wires:
  p/1 -> Demux/1
  eta/1 -> Demux1/1
  Demux/1 -> Terminator1/1
  Demux1/3 -> Cos/1
  Demux1/2 -> Cos1/1, Sin/1
  Demux1/1 -> Terminator2/1
  Demux/2 -> Sum/1
  Constant/1 -> Sum/2
  Demux/3 -> Sum1/1
  Constant1/1 -> Sum1/2
  Sum/1 -> Product/1
  Sin/1 -> Gain1/1, Product/2
  Sum1/1 -> Product1/1
  Cos1/1 -> Vector Concatenate/2, Product1/2
  Product/1 -> Sum2/1
  Product1/1 -> Sum2/2
  Sum2/1 -> Gain/1
  Gain/1 -> Product2/1
  Cos/1 -> Product2/2
  Vector Concatenate/1 -> Transpose/1
  Gain1/1 -> Vector Concatenate/1
  Product2/1 -> Product3/1
  Transpose/1 -> Product3/2
  Product3/1 -> gx/1

== system euler_ZXY_model/CBF-QP(速度入力)/ECBF-QP_rengo_ver./c ==
  p : Inport
  eta : Inport  Port=2
  Cos : Trigonometry  Operator=cos
  Gain : Gain  Gain=alpha/2
  Product : Product
  Selector : Selector  InputPortWidth=3  IndexOptions=Index vector (dialog)  Indices=[3]  OutputSizes=1
  h : Subsystem
  c : Outport
  wires:
  eta/1 -> Selector/1
  p/1 -> h/1(p)
  Selector/1 -> Cos/1
  h/1(h) -> Gain/1
  Gain/1 -> Product/1
  Cos/1 -> Product/2
  Product/1 -> c/1

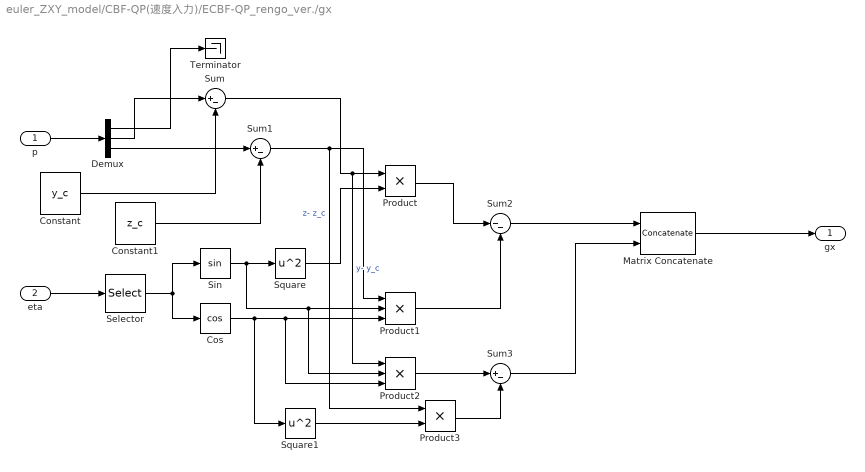
== system euler_ZXY_model/CBF-QP(速度入力)/ECBF-QP_rengo_ver./gx ==
  p : Inport
  eta : Inport  Port=2
  Constant : Constant  Value=y_c
  Constant1 : Constant  Value=z_c
  Cos : Trigonometry  Operator=cos
  Demux : Demux  Outputs=3
  Matrix Concatenate : Concatenate  Mode=Multidimensional array  ConcatenateDimension=2
  Product : Product
  Product1 : Product  Inputs=3
  Product2 : Product  Inputs=3
  Product3 : Product
  Selector : Selector  InputPortWidth=3  IndexOptions=Index vector (dialog)  Indices=[2]  OutputSizes=1
  Sin : Trigonometry
  Square : Math  Operator=square
  Square1 : Math  Operator=square
  Sum : Sum  Inputs=|+-
  Sum1 : Sum  Inputs=|+-
  Sum2 : Sum  Inputs=|--
  Sum3 : Sum  Inputs=|+-
  Terminator : Terminator
  gx : Outport
  wires:
  p/1 -> Demux/1
  Demux/2 -> Sum/1
  Constant/1 -> Sum/2
  Demux/3 -> Sum1/1
  eta/1 -> Selector/1
  Selector/1 -> Sin/1, Cos/1
  Sin/1 -> Product2/2, Product1/2, Square/1
  Square/1 -> Product/2
  Sum/1 -> Product2/1, Product/1  "y- y_c"
  Product/1 -> Sum2/1
  Cos/1 -> Square1/1, Product2/3, Product1/3
  Sum1/1 -> Product3/1, Product1/1  "z- z_c"
  Product1/1 -> Sum2/2
  Sum2/1 -> Matrix Concatenate/1
  Matrix Concatenate/1 -> gx/1
  Product2/1 -> Sum3/1
  Square1/1 -> Product3/2
  Sum3/1 -> Matrix Concatenate/2
  Product3/1 -> Sum3/2
  Constant1/1 -> Sum1/2
  Demux/1 -> Terminator/1

== system euler_ZXY_model/CBF-QP(速度入力)/ECBF-QP_z_only/Subsystem ==
  eta : Inport
  body_velocity : Inport  Port=2
  eta_dot : Inport  Port=3
  Scope : Scope  NumInputPorts=3
  f_x : Subsystem
  fx : Outport
  wires:
  eta/1 -> f_x/1(eta)
  body_velocity/1 -> f_x/2(body_velocity)
  eta_dot/1 -> f_x/3(eta_dot)
  f_x/1(f_x3) -> fx/1, Scope/3

== system euler_ZXY_model/CBF-QP(速度入力)/ECBF-QP_z_only/c ==
  p : Inport
  p_dot : Inport  Port=2
  Gain : Gain  Gain=alpha_1
  Gain1 : Gain  Gain=alpha_2
  Subsystem : Subsystem
  Sum : Sum  Inputs=|++
  h : Subsystem
  c : Outport
  wires:
  p/1 -> h/1(p)
  h/1(h) -> Gain/1
  Gain/1 -> Sum/1
  Sum/1 -> c/1
  Subsystem/1(h_dot) -> Gain1/1
  Gain1/1 -> Sum/2
  p_dot/1 -> Subsystem/1(p_dot)

== system euler_ZXY_model/CBF-QP(速度入力)/ECBF-QP_z_only/gx ==
  eta : Inport
  Cos : Trigonometry  Operator=cos
  Cos1 : Trigonometry  Operator=cos
  Demux1 : Demux  Outputs=3
  Gain1 : Gain  Gain=-1
  Product2 : Product  Inputs=*/
  Product3 : Product
  Sin : Trigonometry
  Terminator2 : Terminator
  Transpose : Math  Operator=transpose
  Vector Concatenate : Concatenate
  gx : Outport
  wires:
  eta/1 -> Demux1/1
  Demux1/3 -> Cos/1
  Demux1/2 -> Cos1/1, Sin/1
  Demux1/1 -> Terminator2/1
  Sin/1 -> Gain1/1
  Cos1/1 -> Product2/1, Vector Concatenate/2
  Cos/1 -> Product2/2
  Vector Concatenate/1 -> Transpose/1
  Gain1/1 -> Vector Concatenate/1
  Product2/1 -> Product3/1
  Transpose/1 -> Product3/2
  Product3/1 -> gx/1

== system euler_ZXY_model/I-CBF(推力修正型)/Euler_matrix_ZXY/Psi_*1 ==
  eta : Inport
  Cos : Trigonometry  Operator=cos
  Cos1 : Trigonometry  Operator=cos
  Demux : Demux  Outputs=3
  Gain : Gain  Gain=-1
  Product : Product
  Product1 : Product
  Sin : Trigonometry
  Sin1 : Trigonometry
  Terminator : Terminator
  Vector Concatenate : Concatenate  NumInputs=3
  Out1 : Outport
  wires:
  eta/1 -> Demux/1
  Demux/1 -> Terminator/1
  Demux/2 -> Cos/1, Sin1/1
  Demux/3 -> Cos1/1, Sin/1
  Cos/1 -> Product1/1, Product/1
  Sin/1 -> Product/2
  Product/1 -> Vector Concatenate/1
  Sin1/1 -> Gain/1
  Gain/1 -> Vector Concatenate/2
  Vector Concatenate/1 -> Out1/1
  Cos1/1 -> Product1/2
  Product1/1 -> Vector Concatenate/3

== system euler_ZXY_model/I-CBF(推力修正型)/Euler_matrix_ZXY/Psi_*2 ==
  eta : Inport
  Constant : Constant  Value=0
  Cos : Trigonometry  Operator=cos
  Demux : Demux  Outputs=3
  Gain : Gain  Gain=-1
  Sin : Trigonometry
  Terminator : Terminator
  Terminator1 : Terminator
  Vector Concatenate : Concatenate  NumInputs=3
  Out1 : Outport
  wires:
  eta/1 -> Demux/1
  Demux/1 -> Terminator/1
  Demux/2 -> Terminator1/1
  Demux/3 -> Sin/1, Cos/1
  Sin/1 -> Gain/1
  Cos/1 -> Vector Concatenate/1
  Constant/1 -> Vector Concatenate/2
  Gain/1 -> Vector Concatenate/3
  Vector Concatenate/1 -> Out1/1

== system euler_ZXY_model/I-CBF(推力修正型)/fx/Elements of Rotation Matrix ==
  R : Inport
  Constant : Constant  Value=e3
  Constant1 : Constant  Value=e2
  Constant2 : Constant  Value=e3
  Display1 : Display
  Display2 : Display
  Matrix Multiply : Product  Multiplication=Matrix(*)
  Matrix Multiply1 : Product  Multiplication=Matrix(*)
  Matrix Multiply2 : Product  Multiplication=Matrix(*)
  Mux : Mux  Inputs=2
  Transpose : Math  Operator=transpose
  Transpose1 : Math  Operator=transpose
  r_32 : Outport
  r_33 : Outport  Port=2
  wires:
  Constant/1 -> Matrix Multiply/2
  R/1 -> Display2/1, Matrix Multiply/1
  Constant1/1 -> Transpose/1
  Transpose/1 -> Matrix Multiply1/1
  Matrix Multiply/1 -> Matrix Multiply2/2, Matrix Multiply1/2
  Matrix Multiply1/1 -> Mux/1, r_32/1
  Matrix Multiply2/1 -> Mux/2, r_33/1
  Constant2/1 -> Transpose1/1
  Transpose1/1 -> Matrix Multiply2/1
  Mux/1 -> Display1/1

== system euler_ZXY_model/I-CBF(推力修正型)/gx/Elements of Rotation Matrix ==
  R : Inport
  Constant : Constant  Value=e3
  Constant2 : Constant  Value=e3
  Display2 : Display
  Matrix Multiply : Product  Multiplication=Matrix(*)
  Matrix Multiply1 : Product  Multiplication=Matrix(*)
  Transpose1 : Math  Operator=transpose
  r_33 : Outport
  wires:
  Constant/1 -> Matrix Multiply/2
  R/1 -> Display2/1, Matrix Multiply/1
  Matrix Multiply1/1 -> r_33/1
  Constant2/1 -> Transpose1/1
  Matrix Multiply/1 -> Matrix Multiply1/2
  Transpose1/1 -> Matrix Multiply1/1

== system euler_ZXY_model/Velocity Feedback Controller/Euler_matrix_ZXY/Psi_*1 ==
  eta : Inport
  Cos : Trigonometry  Operator=cos
  Cos1 : Trigonometry  Operator=cos
  Demux : Demux  Outputs=3
  Gain : Gain  Gain=-1
  Product : Product
  Product1 : Product
  Sin : Trigonometry
  Sin1 : Trigonometry
  Terminator : Terminator
  Vector Concatenate : Concatenate  NumInputs=3
  Out1 : Outport
  wires:
  eta/1 -> Demux/1
  Demux/1 -> Terminator/1
  Demux/2 -> Cos/1, Sin1/1
  Demux/3 -> Cos1/1, Sin/1
  Cos/1 -> Product1/1, Product/1
  Sin/1 -> Product/2
  Product/1 -> Vector Concatenate/1
  Sin1/1 -> Gain/1
  Gain/1 -> Vector Concatenate/2
  Vector Concatenate/1 -> Out1/1
  Cos1/1 -> Product1/2
  Product1/1 -> Vector Concatenate/3

== system euler_ZXY_model/Velocity Feedback Controller/Euler_matrix_ZXY/Psi_*2 ==
  eta : Inport
  Constant : Constant  Value=0
  Cos : Trigonometry  Operator=cos
  Demux : Demux  Outputs=3
  Gain : Gain  Gain=-1
  Sin : Trigonometry
  Terminator : Terminator
  Terminator1 : Terminator
  Vector Concatenate : Concatenate  NumInputs=3
  Out1 : Outport
  wires:
  eta/1 -> Demux/1
  Demux/1 -> Terminator/1
  Demux/2 -> Terminator1/1
  Demux/3 -> Sin/1, Cos/1
  Sin/1 -> Gain/1
  Cos/1 -> Vector Concatenate/1
  Constant/1 -> Vector Concatenate/2
  Gain/1 -> Vector Concatenate/3
  Vector Concatenate/1 -> Out1/1

== system euler_ZXY_model/dynamics/並進方向の運動方程式/B ==
  R : Inport
  Constant : Constant  Value=e1
  Matrix Concatenate : Concatenate  Mode=Multidimensional array
  Subsystem : Subsystem
  Transpose1 : Math  Operator=transpose
  B : Outport
  A : Outport  Port=2
  wires:
  Constant/1 -> Transpose1/1
  Matrix Concatenate/1 -> B/1  "B"
  Subsystem/1(A) -> Matrix Concatenate/1, A/1  "A"
  R/1 -> Subsystem/1(R)
  Transpose1/1 -> Matrix Concatenate/2

== system euler_ZXY_model/dynamics/並進方向の運動方程式/Rotation matrix_ZXY ==
  eta : Inport
  Matrix Concatenate : Concatenate  NumInputs=3  Mode=Multidimensional array  ConcatenateDimension=2
  R1 : Subsystem
  R2 : Subsystem
  R3 : Subsystem
  R : Outport  VectorParamsAs1DForOutWhenUnconnected=off
  wires:
  eta/1 -> R1/1(In1), R3/1(In1), R2/1(In1)
  R3/1(Out1) -> Matrix Concatenate/3
  R2/1(Out1) -> Matrix Concatenate/2
  R1/1(Out1) -> Matrix Concatenate/1
  Matrix Concatenate/1 -> R/1

== system euler_ZXY_model/dynamics/並進方向の運動方程式/To workspace ==
  xi_wb : Inport
  Clock : Clock
  Selector : Selector  InputPortWidth=3  IndexOptions=Index vector (dialog)  Indices=1  OutputSizes=1
  Selector1 : Selector  InputPortWidth=3  IndexOptions=Index vector (dialog)  Indices=2  OutputSizes=1
  Selector2 : Selector  InputPortWidth=3  IndexOptions=Index vector (dialog)  Indices=3  OutputSizes=1
  To Workspace1 : ToWorkspace  VariableName=drone_ySm  SampleTime=-1
      settings: Save2DSignal=2-D array (concatenate along first dimension)
  To Workspace10 : ToWorkspace  VariableName=drone_xSm  SampleTime=-1
      settings: Save2DSignal=2-D array (concatenate along first dimension)
  To Workspace2 : ToWorkspace  VariableName=drone_zSm  SampleTime=-1
      settings: Save2DSignal=2-D array (concatenate along first dimension)
  To Workspace8 : ToWorkspace  VariableName=time  SampleTime=-1
      settings: Save2DSignal=2-D array (concatenate along first dimension)
  wires:
  xi_wb/1 -> Selector2/1, Selector1/1, Selector/1
  Selector/1 -> To Workspace10/1
  Selector2/1 -> To Workspace2/1
  Selector1/1 -> To Workspace1/1
  Clock/1 -> To Workspace8/1

== system euler_ZXY_model/dynamics/並進方向の運動方程式/lambda1,lambda3 ==
  note: $[\lambda_1 ~ \lambda_3 ]^T = (BB^T)^{-1} (BRF^b - mgBe_3 + m\dot{B}\dot{p})$
  p_dot : Inport
  mge_3 : Inport  Port=2
  RF^b : Inport  Port=3
  B : Inport  Port=4
  Add : Sum  Inputs=+-+
  Derivative : Derivative
  Divide2 : Product  Inputs=/*  Multiplication=Matrix(*)
  Gain : Gain  Gain=m
  MatrixMultiply{,1..3} (4 alike) : Product  Multiplication=Matrix(*)
  Transpose : Math  Operator=transpose
  "[lambda_1 lambda_2]^T" : Outport
  wires:
  B/1 -> Derivative/1, MatrixMultiply1/1, MatrixMultiply/1, Transpose/1, MatrixMultiply3/1
  Divide2/1 -> "[lambda_1 lambda_2]^T"/1
  p_dot/1 -> MatrixMultiply2/2
  MatrixMultiply3/1 -> Divide2/1
  MatrixMultiply1/1 -> Add/2
  MatrixMultiply2/1 -> Gain/1
  Derivative/1 -> MatrixMultiply2/1
  RF^b/1 -> MatrixMultiply/2
  Transpose/1 -> MatrixMultiply3/2
  mge_3/1 -> MatrixMultiply1/2
  MatrixMultiply/1 -> Add/1
  Gain/1 -> Add/3
  Add/1 -> Divide2/2

== system euler_ZXY_model/dynamics/回転方向の運動方程式/C(η,η_dot) ==
  Ψ(η) : Inport
  eta_dot : Inport  Port=2
  Constant : Constant  Value=J  VectorParams1D=off
  Constant1 : Constant  Value=J  VectorParams1D=off
  Derivative : Derivative
  Math Function : Math  Operator=transpose  SignedPower=on
  Math Function1 : Math  Operator=transpose  SignedPower=on
  Product : Product  Inputs=4  Multiplication=Matrix(*)
  Product1 : Product  Inputs=3  Multiplication=Matrix(*)
  Sum : Sum
  skew : Subsystem
  C(eta,deta) : Outport  VectorParamsAs1DForOutWhenUnconnected=off
  tag scope: C=global
  wires:
  Derivative/1 -> Product1/3
  Product/1 -> Sum/2
  Sum/1 -> C(eta,deta)/1, [C]
  Math Function1/1 -> Product1/1
  Ψ(η)/1 -> Math Function1/1, Derivative/1, Product/4, Math Function/1, skew/1(Ψ(η))
  Product1/1 -> Sum/1
  Constant1/1 -> Product1/2
  eta_dot/1 -> skew/2(eta_dot)
  Math Function/1 -> Product/1
  skew/1(skew(Ω)) -> Product/2
  Constant/1 -> Product/3

== system euler_ZXY_model/dynamics/回転方向の運動方程式/Euler_matrix_ZXY ==
  eta : Inport
  Constant : Constant  Value=e2
  Matrix Concatenate4 : Concatenate  NumInputs=3  Mode=Multidimensional array  ConcatenateDimension=2
  Psi_*1 : Subsystem
  Psi_*2 : Subsystem
  オイラー角逆行列Ψ(η) : Outport  VectorParamsAs1DForOutWhenUnconnected=off
  wires:
  eta/1 -> Psi_*1/1(eta), Psi_*2/1(eta)
  Matrix Concatenate4/1 -> オイラー角逆行列Ψ(η)/1
  Psi_*2/1(Out1) -> Matrix Concatenate4/2
  Psi_*1/1(Out1) -> Matrix Concatenate4/1
  Constant/1 -> Matrix Concatenate4/3

== system euler_ZXY_model/dynamics/回転方向の運動方程式/M(η)の算出 ==
  Ψ(η) : Inport
  Constant : Constant  Value=J  VectorParams1D=off
  Math Function1 : Math  Operator=transpose  SignedPower=on
  Product : Product  Inputs=3  Multiplication=Matrix(*)
  M(η) : Outport  VectorParamsAs1DForOutWhenUnconnected=off
  wires:
  Math Function1/1 -> Product/1
  Ψ(η)/1 -> Math Function1/1, Product/3
  Constant/1 -> Product/2
  Product/1 -> M(η)/1

== system euler_ZXY_model/dynamics/回転方向の運動方程式/Rotation matrix_ZXY ==
  eta : Inport
  Matrix Concatenate : Concatenate  NumInputs=3  Mode=Multidimensional array  ConcatenateDimension=2
  R1 : Subsystem
  R2 : Subsystem
  R3 : Subsystem
  R : Outport  VectorParamsAs1DForOutWhenUnconnected=off
  wires:
  eta/1 -> R1/1(In1), R3/1(In1), R2/1(In1)
  R3/1(Out1) -> Matrix Concatenate/3
  R2/1(Out1) -> Matrix Concatenate/2
  R1/1(Out1) -> Matrix Concatenate/1
  Matrix Concatenate/1 -> R/1
